simulink model "simulinkm2"  (R2020b)
settings: Solver=VariableStepAuto  StartTime=0.0  StopTime=10.0  RelTol=1e-3
(part 4 of 5)

== matlab function simulinkm2/MATLAB Function3 ==
  data: q input; A_F output; q_dot input; q_double_dot input
  function A_F = forward_acceleration_kinematics(q,q_dot, q_double_dot)
  
     q1 = q(1)
     q2 = q(2)
     q3 = q(3)
     q4 = q(4)
     q5 = q(5)
     q6 = q(6)
     q_double_dot1 = q_double_dot(1) 
     q_double_dot2 = q_double_dot(2) 
     q_double_dot3 = q_double_dot(3) 
     q_double_dot4 = q_double_dot(4) 
     q_double_dot5 = q_double_dot(5) 
     q_double_dot6 = q_double_dot(6)
     q_dot1 = q_dot(1)
     q_dot2 = q_dot(2)
     q_dot3 = q_dot(3)
     q_dot4 = q_dot(4)
     q_dot5 = q_dot(5)
     q_dot6 = q_dot(6)
  
   j_dot = [-q_dot1*((pi*cos((pi*q1)/180))/36 + 10*sin((pi*q5)/180)*((pi*sin((pi*q1)/180)*sin((pi*q4)/180))/180 + (pi*cos((pi*q1)/180)*cos((pi*q2)/180)*cos((pi*q3)/180)*cos((pi*q4)/180))/180 - (pi*cos((pi*q1)/180)*cos((pi*q4)/180)*sin((pi*q2)/180)*sin((pi*q3)/180))/180) + (pi*cos((pi*q1)/180)*cos((pi*q2)/180))/36 + (pi*sin((pi*(q2 + q3))/180)*cos((pi*q1)/180)*cos((pi*q5)/180))/18 + (pi*cos((pi*q1)/180)*cos((pi*q2)/180)*sin((pi*q3)/180))/18 + (pi*cos((pi*q1)/180)*cos((pi*q3)/180)*sin((pi*q2)/180))/18),                                                                                                                                                                                                                                                                                                                                                                                                                                                                                                                                                                                                                                              -q_dot2*cos((pi*q1)/180)*((pi*sin((pi*(q2 + q3))/180))/18 + (pi*cos((pi*q2)/180))/36 + (pi*cos((pi*(q2 + q3))/180)*sin((pi*(q4 + q5))/180))/36 + (pi*sin((pi*(q2 + q3))/180)*cos((pi*q5)/180))/18 - (pi*cos((pi*(q2 + q3))/180)*sin((pi*(q4 - q5))/180))/36),                                                                                                                                                                                                                                                                                                                                                                                                                                                                                                                                                                                 -q_dot3*cos((pi*q1)/180)*((pi*sin((pi*(q2 + q3))/180))/18 + (pi*cos((pi*(q2 + q3))/180)*sin((pi*(q4 + q5))/180))/36 + (pi*sin((pi*(q2 + q3))/180)*cos((pi*q5)/180))/18 - (pi*cos((pi*(q2 + q3))/180)*sin((pi*(q4 - q5))/180))/36),                                                                                                                             -q_dot4*(10*cos((pi*(q2 + q3))/180)*sin((pi*q5)/180)*((pi*cos((pi*q1)/180)*cos((pi*q4)/180))/180 - (pi*sin((pi*q1)/180)*sin((pi*q2)/180)*sin((pi*q3)/180)*sin((pi*q4)/180))/180 + (pi*cos((pi*q2)/180)*cos((pi*q3)/180)*sin((pi*q1)/180)*sin((pi*q4)/180))/180) - sin((pi*(q2 + q3))/180)*sin((pi*q1)/180)*((pi*cos((pi*(q4 + q5))/180)*sin((pi*(q2 + q3))/180))/36 - (pi*sin((pi*(q2 + q3))/180)*cos((pi*(q4 - q5))/180))/36)),                                                                                                                                                                                                                                -q_dot5*((cos((pi*q1)/180)*cos((pi*q4)/180) - sin((pi*q4)/180)*(sin((pi*q1)/180)*sin((pi*q2)/180)*sin((pi*q3)/180) - cos((pi*q2)/180)*cos((pi*q3)/180)*sin((pi*q1)/180)))*((pi*cos((pi*(q4 + q5))/180)*sin((pi*(q2 + q3))/180))/36 + (pi*cos((pi*(q2 + q3))/180)*sin((pi*q5)/180))/18 + (pi*sin((pi*(q2 + q3))/180)*cos((pi*(q4 - q5))/180))/36) + sin((pi*(q2 + q3))/180)*sin((pi*q4)/180)*((pi*cos((pi*q5)/180)*(cos((pi*q1)/180)*sin((pi*q4)/180) - cos((pi*q2)/180)*cos((pi*q3)/180)*cos((pi*q4)/180)*sin((pi*q1)/180) + cos((pi*q4)/180)*sin((pi*q1)/180)*sin((pi*q2)/180)*sin((pi*q3)/180)))/18 + (pi*sin((pi*(q2 + q3))/180)*sin((pi*q1)/180)*sin((pi*q5)/180))/18)), 0;
                   -q_dot1*((pi*sin((pi*q1)/180))/36 - 10*sin((pi*q5)/180)*((pi*cos((pi*q1)/180)*sin((pi*q4)/180))/180 - (pi*cos((pi*q2)/180)*cos((pi*q3)/180)*cos((pi*q4)/180)*sin((pi*q1)/180))/180 + (pi*cos((pi*q4)/180)*sin((pi*q1)/180)*sin((pi*q2)/180)*sin((pi*q3)/180))/180) + (pi*cos((pi*q2)/180)*sin((pi*q1)/180))/36 + (pi*sin((pi*(q2 + q3))/180)*cos((pi*q5)/180)*sin((pi*q1)/180))/18 + (pi*cos((pi*q2)/180)*sin((pi*q1)/180)*sin((pi*q3)/180))/18 + (pi*cos((pi*q3)/180)*sin((pi*q1)/180)*sin((pi*q2)/180))/18),                                                                                                                                                                                                                                                                                                                                                                                                                                                                                                                                                                                                                                              -q_dot2*sin((pi*q1)/180)*((pi*sin((pi*(q2 + q3))/180))/18 + (pi*cos((pi*q2)/180))/36 + (pi*cos((pi*(q2 + q3))/180)*sin((pi*(q4 + q5))/180))/36 + (pi*sin((pi*(q2 + q3))/180)*cos((pi*q5)/180))/18 - (pi*cos((pi*(q2 + q3))/180)*sin((pi*(q4 - q5))/180))/36),                                                                                                                                                                                                                                                                                                                                                                                                                                                                                                                                                                                 -q_dot3*sin((pi*q1)/180)*((pi*sin((pi*(q2 + q3))/180))/18 + (pi*cos((pi*(q2 + q3))/180)*sin((pi*(q4 + q5))/180))/36 + (pi*sin((pi*(q2 + q3))/180)*cos((pi*q5)/180))/18 - (pi*cos((pi*(q2 + q3))/180)*sin((pi*(q4 - q5))/180))/36),                                                                                                                             -q_dot4*(10*cos((pi*(q2 + q3))/180)*sin((pi*q5)/180)*((pi*cos((pi*q4)/180)*sin((pi*q1)/180))/180 - (pi*cos((pi*q1)/180)*cos((pi*q2)/180)*cos((pi*q3)/180)*sin((pi*q4)/180))/180 + (pi*cos((pi*q1)/180)*sin((pi*q2)/180)*sin((pi*q3)/180)*sin((pi*q4)/180))/180) + sin((pi*(q2 + q3))/180)*cos((pi*q1)/180)*((pi*cos((pi*(q4 + q5))/180)*sin((pi*(q2 + q3))/180))/36 - (pi*sin((pi*(q2 + q3))/180)*cos((pi*(q4 - q5))/180))/36)),                                                                                                                                                                                                                                -q_dot5*((sin((pi*q4)/180)*(cos((pi*q1)/180)*sin((pi*q2)/180)*sin((pi*q3)/180) - cos((pi*q1)/180)*cos((pi*q2)/180)*cos((pi*q3)/180)) + cos((pi*q4)/180)*sin((pi*q1)/180))*((pi*cos((pi*(q4 + q5))/180)*sin((pi*(q2 + q3))/180))/36 + (pi*cos((pi*(q2 + q3))/180)*sin((pi*q5)/180))/18 + (pi*sin((pi*(q2 + q3))/180)*cos((pi*(q4 - q5))/180))/36) + sin((pi*(q2 + q3))/180)*sin((pi*q4)/180)*((pi*cos((pi*q5)/180)*(sin((pi*q1)/180)*sin((pi*q4)/180) + cos((pi*q1)/180)*cos((pi*q2)/180)*cos((pi*q3)/180)*cos((pi*q4)/180) - cos((pi*q1)/180)*cos((pi*q4)/180)*sin((pi*q2)/180)*sin((pi*q3)/180)))/18 - (pi*sin((pi*(q2 + q3))/180)*cos((pi*q1)/180)*sin((pi*q5)/180))/18)), 0;
                                                                                                                                                                                                                                                                                                                                                                                                                                                                                                                               0, -q_dot2*(sin((pi*q1)/180)*(10*sin((pi*q5)/180)*((pi*cos((pi*q2)/180)*cos((pi*q4)/180)*sin((pi*q1)/180)*sin((pi*q3)/180))/180 + (pi*cos((pi*q3)/180)*cos((pi*q4)/180)*sin((pi*q1)/180)*sin((pi*q2)/180))/180) + (pi*sin((pi*q1)/180)*sin((pi*q2)/180))/36 - (pi*cos((pi*(q2 + q3))/180)*cos((pi*q5)/180)*sin((pi*q1)/180))/18 - (pi*cos((pi*q2)/180)*cos((pi*q3)/180)*sin((pi*q1)/180))/18 + (pi*sin((pi*q1)/180)*sin((pi*q2)/180)*sin((pi*q3)/180))/18) + cos((pi*q1)/180)*(10*sin((pi*q5)/180)*((pi*cos((pi*q1)/180)*cos((pi*q2)/180)*cos((pi*q4)/180)*sin((pi*q3)/180))/180 + (pi*cos((pi*q1)/180)*cos((pi*q3)/180)*cos((pi*q4)/180)*sin((pi*q2)/180))/180) + (pi*cos((pi*q1)/180)*sin((pi*q2)/180))/36 - (pi*cos((pi*(q2 + q3))/180)*cos((pi*q1)/180)*cos((pi*q5)/180))/18 - (pi*cos((pi*q1)/180)*cos((pi*q2)/180)*cos((pi*q3)/180))/18 + (pi*cos((pi*q1)/180)*sin((pi*q2)/180)*sin((pi*q3)/180))/18)), -q_dot3*(sin((pi*q1)/180)*(10*sin((pi*q5)/180)*((pi*cos((pi*q2)/180)*cos((pi*q4)/180)*sin((pi*q1)/180)*sin((pi*q3)/180))/180 + (pi*cos((pi*q3)/180)*cos((pi*q4)/180)*sin((pi*q1)/180)*sin((pi*q2)/180))/180) - (pi*cos((pi*(q2 + q3))/180)*cos((pi*q5)/180)*sin((pi*q1)/180))/18 - (pi*cos((pi*q2)/180)*cos((pi*q3)/180)*sin((pi*q1)/180))/18 + (pi*sin((pi*q1)/180)*sin((pi*q2)/180)*sin((pi*q3)/180))/18) + cos((pi*q1)/180)*(10*sin((pi*q5)/180)*((pi*cos((pi*q1)/180)*cos((pi*q2)/180)*cos((pi*q4)/180)*sin((pi*q3)/180))/180 + (pi*cos((pi*q1)/180)*cos((pi*q3)/180)*cos((pi*q4)/180)*sin((pi*q2)/180))/180) - (pi*cos((pi*(q2 + q3))/180)*cos((pi*q1)/180)*cos((pi*q5)/180))/18 - (pi*cos((pi*q1)/180)*cos((pi*q2)/180)*cos((pi*q3)/180))/18 + (pi*cos((pi*q1)/180)*sin((pi*q2)/180)*sin((pi*q3)/180))/18)), -q_dot4*(10*sin((pi*(q2 + q3))/180)*cos((pi*q1)/180)*sin((pi*q5)/180)*((pi*cos((pi*q1)/180)*cos((pi*q4)/180))/180 - (pi*sin((pi*q1)/180)*sin((pi*q2)/180)*sin((pi*q3)/180)*sin((pi*q4)/180))/180 + (pi*cos((pi*q2)/180)*cos((pi*q3)/180)*sin((pi*q1)/180)*sin((pi*q4)/180))/180) + 10*sin((pi*(q2 + q3))/180)*sin((pi*q1)/180)*sin((pi*q5)/180)*((pi*cos((pi*q4)/180)*sin((pi*q1)/180))/180 - (pi*cos((pi*q1)/180)*cos((pi*q2)/180)*cos((pi*q3)/180)*sin((pi*q4)/180))/180 + (pi*cos((pi*q1)/180)*sin((pi*q2)/180)*sin((pi*q3)/180)*sin((pi*q4)/180))/180)), q_dot5*((cos((pi*q1)/180)*cos((pi*q4)/180) - sin((pi*q4)/180)*(sin((pi*q1)/180)*sin((pi*q2)/180)*sin((pi*q3)/180) - cos((pi*q2)/180)*cos((pi*q3)/180)*sin((pi*q1)/180)))*((pi*cos((pi*q5)/180)*(sin((pi*q1)/180)*sin((pi*q4)/180) + cos((pi*q1)/180)*cos((pi*q2)/180)*cos((pi*q3)/180)*cos((pi*q4)/180) - cos((pi*q1)/180)*cos((pi*q4)/180)*sin((pi*q2)/180)*sin((pi*q3)/180)))/18 - (pi*sin((pi*(q2 + q3))/180)*cos((pi*q1)/180)*sin((pi*q5)/180))/18) - (sin((pi*q4)/180)*(cos((pi*q1)/180)*sin((pi*q2)/180)*sin((pi*q3)/180) - cos((pi*q1)/180)*cos((pi*q2)/180)*cos((pi*q3)/180)) + cos((pi*q4)/180)*sin((pi*q1)/180))*((pi*cos((pi*q5)/180)*(cos((pi*q1)/180)*sin((pi*q4)/180) - cos((pi*q2)/180)*cos((pi*q3)/180)*cos((pi*q4)/180)*sin((pi*q1)/180) + cos((pi*q4)/180)*sin((pi*q1)/180)*sin((pi*q2)/180)*sin((pi*q3)/180)))/18 + (pi*sin((pi*(q2 + q3))/180)*sin((pi*q1)/180)*sin((pi*q5)/180))/18)), 0;
                                                                                                                                                                                                                                                                                                                                                                                                                                                                                                                               0,                                                                                                                                                                                                                                                                                                                                                                                                                                                                                                                                                                                                                                                                                                                                                                                                                                                                                                         0,                                                                                                                                                                                                                                                                                                                                                                                                                                                                                                                                                                                                                                                                                                                                                                                                                 0,                                                                                                                                                                                                                                                                                                                                                                                                                                                                                                                                                           0,                                                                                                                                                                                                                                                                                                                                                                                                                                                                                                                                                                                                                                                                                                                                                                                                                                                                                                          0, 0;
                                                                                                                                                                                                                                                                                                                                                                                                                                                                                                                               0,                                                                                                                                                                                                                                                                                                                                                                                                                                                                                                                                                                                                                                                                                                                                                                                                                                                                                                         0,                                                                                                                                                                                                                                                                                                                                                                                                                                                                                                                                                                                                                                                                                                                                                                                                                 0,                                                                                                                                                                                                                                                                                                                                                                                                                                                                                                                                                           0,                                                                                                                                                                                                                                                                                                                                                                                                                                                                                                                                                                                                                                                                                                                                                                                                                                                                                                          0, 0;
                                                                                                                                                                                                                                                                                                                                                                                                                                                                                                                               0,                                                                                                                                                                                                                                                                                                                                                                                                                                                                                                                                                                                                                                                                                                                                                                                                                                                                                                         0,                                                                                                                                                                                                                                                                                                                                                                                                                                                                                                                                                                                                                                                                                                                                                                                                                 0,                                                                                                                                                                                                                                                                                                                                                                                                                                                                                                                                                           0,                                                                                                                                                                                                                                                                                                                                                                                                                                                                                                                                                                                                                                                                                                                                                                                                                                                                                                          0, 0]
                                      
   J =[10*sin((pi*q5)/180)*(cos((pi*q1)/180)*sin((pi*q4)/180) - cos((pi*q2)/180)*cos((pi*q3)/180)*cos((pi*q4)/180)*sin((pi*q1)/180) + cos((pi*q4)/180)*sin((pi*q1)/180)*sin((pi*q2)/180)*sin((pi*q3)/180)) - 5*cos((pi*q2)/180)*sin((pi*q1)/180) - 5*sin((pi*q1)/180) - 10*cos((pi*q2)/180)*sin((pi*q1)/180)*sin((pi*q3)/180) - 10*cos((pi*q3)/180)*sin((pi*q1)/180)*sin((pi*q2)/180) - 10*sin((pi*(q2 + q3))/180)*cos((pi*q5)/180)*sin((pi*q1)/180),                                                                                                                                                                                                                                                                                                                                                                                                                                                                                                                                                                                                                                                                  cos((pi*q1)/180)*(10*cos((pi*(q2 + q3))/180) - 5*sin((pi*q2)/180) - 5*sin((pi*(q2 + q3))/180)*sin((pi*(q4 + q5))/180) + 10*cos((pi*(q2 + q3))/180)*cos((pi*q5)/180) + 5*sin((pi*(q2 + q3))/180)*sin((pi*(q4 - q5))/180)),                                                                                                                                                                                                                                                                                                                                                                                                                                                                                                                                                                                                                                                                                                                                                                                                                         cos((pi*q1)/180)*(10*cos((pi*(q2 + q3))/180) - 5*sin((pi*(q2 + q3))/180)*sin((pi*(q4 + q5))/180) + 10*cos((pi*(q2 + q3))/180)*cos((pi*q5)/180) + 5*sin((pi*(q2 + q3))/180)*sin((pi*(q4 - q5))/180)),                                                                                                                                                                                                                                                                                                                           cos((pi*(q2 + q3))/180)*(5*sin((pi*q1)/180) + 5*cos((pi*q2)/180)*sin((pi*q1)/180) - 5*sin((pi*q1)/180)*(cos((pi*q2)/180) + 1) - 10*sin((pi*q5)/180)*(cos((pi*q1)/180)*sin((pi*q4)/180) - cos((pi*q2)/180)*cos((pi*q3)/180)*cos((pi*q4)/180)*sin((pi*q1)/180) + cos((pi*q4)/180)*sin((pi*q1)/180)*sin((pi*q2)/180)*sin((pi*q3)/180)) + 10*cos((pi*q2)/180)*sin((pi*q1)/180)*sin((pi*q3)/180) + 10*cos((pi*q3)/180)*sin((pi*q1)/180)*sin((pi*q2)/180) + 10*sin((pi*(q2 + q3))/180)*cos((pi*q5)/180)*sin((pi*q1)/180)) - sin((pi*(q2 + q3))/180)*sin((pi*q1)/180)*(10*cos((pi*(q2 + q3))/180) - 5*sin((pi*(q2 + q3))/180)*sin((pi*(q4 + q5))/180) + 10*cos((pi*(q2 + q3))/180)*cos((pi*q5)/180) + 5*sin((pi*(q2 + q3))/180)*sin((pi*(q4 - q5))/180)),                                                                                                                                                                                                                                                                                                                                                                                                                                                                                           (cos((pi*q1)/180)*cos((pi*q4)/180) - sin((pi*q4)/180)*(sin((pi*q1)/180)*sin((pi*q2)/180)*sin((pi*q3)/180) - cos((pi*q2)/180)*cos((pi*q3)/180)*sin((pi*q1)/180)))*(10*cos((pi*(q2 + q3))/180)*cos((pi*q5)/180) - 5*sin((pi*(q2 + q3))/180)*sin((pi*(q4 + q5))/180) + 5*sin((pi*(q2 + q3))/180)*sin((pi*(q4 - q5))/180)) + sin((pi*(q2 + q3))/180)*sin((pi*q4)/180)*(5*sin((pi*q1)/180) + 5*cos((pi*q2)/180)*sin((pi*q1)/180) - 5*sin((pi*q1)/180)*(2*sin((pi*(q2 + q3))/180) + cos((pi*q2)/180) + 1) - 10*sin((pi*q5)/180)*(cos((pi*q1)/180)*sin((pi*q4)/180) - cos((pi*q2)/180)*cos((pi*q3)/180)*cos((pi*q4)/180)*sin((pi*q1)/180) + cos((pi*q4)/180)*sin((pi*q1)/180)*sin((pi*q2)/180)*sin((pi*q3)/180)) + 10*cos((pi*q2)/180)*sin((pi*q1)/180)*sin((pi*q3)/180) + 10*cos((pi*q3)/180)*sin((pi*q1)/180)*sin((pi*q2)/180) + 10*sin((pi*(q2 + q3))/180)*cos((pi*q5)/180)*sin((pi*q1)/180)),                                                                                                                                                                                                                                                                                                                                                                                                                                                                                                                                                                             (cos((pi*(q2 + q3))/180)*cos((pi*q5)/180) - sin((pi*(q2 + q3))/180)*cos((pi*q4)/180)*sin((pi*q5)/180))*(5*sin((pi*q1)/180) + 5*cos((pi*q2)/180)*sin((pi*q1)/180) - 5*sin((pi*q1)/180)*(2*sin((pi*(q2 + q3))/180) + cos((pi*q2)/180) + 1) - 10*sin((pi*q5)/180)*(cos((pi*q1)/180)*sin((pi*q4)/180) - cos((pi*q2)/180)*cos((pi*q3)/180)*cos((pi*q4)/180)*sin((pi*q1)/180) + cos((pi*q4)/180)*sin((pi*q1)/180)*sin((pi*q2)/180)*sin((pi*q3)/180)) + 10*cos((pi*q2)/180)*sin((pi*q1)/180)*sin((pi*q3)/180) + 10*cos((pi*q3)/180)*sin((pi*q1)/180)*sin((pi*q2)/180) + 10*sin((pi*(q2 + q3))/180)*cos((pi*q5)/180)*sin((pi*q1)/180)) + (sin((pi*q5)/180)*(cos((pi*q4)/180)*(sin((pi*q1)/180)*sin((pi*q2)/180)*sin((pi*q3)/180) - cos((pi*q2)/180)*cos((pi*q3)/180)*sin((pi*q1)/180)) + cos((pi*q1)/180)*sin((pi*q4)/180)) - cos((pi*q5)/180)*(cos((pi*q2)/180)*sin((pi*q1)/180)*sin((pi*q3)/180) + cos((pi*q3)/180)*sin((pi*q1)/180)*sin((pi*q2)/180)))*(10*cos((pi*(q2 + q3))/180)*cos((pi*q5)/180) - 5*sin((pi*(q2 + q3))/180)*sin((pi*(q4 + q5))/180) + 5*sin((pi*(q2 + q3))/180)*sin((pi*(q4 - q5))/180));
5*cos((pi*q1)/180) + 5*cos((pi*q1)/180)*cos((pi*q2)/180) + 10*sin((pi*q5)/180)*(sin((pi*q1)/180)*sin((pi*q4)/180) + cos((pi*q1)/180)*cos((pi*q2)/180)*cos((pi*q3)/180)*cos((pi*q4)/180) - cos((pi*q1)/180)*cos((pi*q4)/180)*sin((pi*q2)/180)*sin((pi*q3)/180)) + 10*sin((pi*(q2 + q3))/180)*cos((pi*q1)/180)*cos((pi*q5)/180) + 10*cos((pi*q1)/180)*cos((pi*q2)/180)*sin((pi*q3)/180) + 10*cos((pi*q1)/180)*cos((pi*q3)/180)*sin((pi*q2)/180),                                                                                                                                                                                                                                                                                                                                                                                                                                                                                                                                                                                                                                                                  sin((pi*q1)/180)*(10*cos((pi*(q2 + q3))/180) - 5*sin((pi*q2)/180) - 5*sin((pi*(q2 + q3))/180)*sin((pi*(q4 + q5))/180) + 10*cos((pi*(q2 + q3))/180)*cos((pi*q5)/180) + 5*sin((pi*(q2 + q3))/180)*sin((pi*(q4 - q5))/180)),                                                                                                                                                                                                                                                                                                                                                                                                                                                                                                                                                                                                                                                                                                                                                                                                                         sin((pi*q1)/180)*(10*cos((pi*(q2 + q3))/180) - 5*sin((pi*(q2 + q3))/180)*sin((pi*(q4 + q5))/180) + 10*cos((pi*(q2 + q3))/180)*cos((pi*q5)/180) + 5*sin((pi*(q2 + q3))/180)*sin((pi*(q4 - q5))/180)),                                                                                                                                                                                                                                                                                                                           sin((pi*(q2 + q3))/180)*cos((pi*q1)/180)*(10*cos((pi*(q2 + q3))/180) - 5*sin((pi*(q2 + q3))/180)*sin((pi*(q4 + q5))/180) + 10*cos((pi*(q2 + q3))/180)*cos((pi*q5)/180) + 5*sin((pi*(q2 + q3))/180)*sin((pi*(q4 - q5))/180)) - cos((pi*(q2 + q3))/180)*(5*cos((pi*q1)/180) + 5*cos((pi*q1)/180)*cos((pi*q2)/180) - 5*cos((pi*q1)/180)*(cos((pi*q2)/180) + 1) + 10*sin((pi*q5)/180)*(sin((pi*q1)/180)*sin((pi*q4)/180) + cos((pi*q1)/180)*cos((pi*q2)/180)*cos((pi*q3)/180)*cos((pi*q4)/180) - cos((pi*q1)/180)*cos((pi*q4)/180)*sin((pi*q2)/180)*sin((pi*q3)/180)) + 10*sin((pi*(q2 + q3))/180)*cos((pi*q1)/180)*cos((pi*q5)/180) + 10*cos((pi*q1)/180)*cos((pi*q2)/180)*sin((pi*q3)/180) + 10*cos((pi*q1)/180)*cos((pi*q3)/180)*sin((pi*q2)/180)),                                                                                                                                                                                                                                                                                                                                                                                                                                                                                           (sin((pi*q4)/180)*(cos((pi*q1)/180)*sin((pi*q2)/180)*sin((pi*q3)/180) - cos((pi*q1)/180)*cos((pi*q2)/180)*cos((pi*q3)/180)) + cos((pi*q4)/180)*sin((pi*q1)/180))*(10*cos((pi*(q2 + q3))/180)*cos((pi*q5)/180) - 5*sin((pi*(q2 + q3))/180)*sin((pi*(q4 + q5))/180) + 5*sin((pi*(q2 + q3))/180)*sin((pi*(q4 - q5))/180)) - sin((pi*(q2 + q3))/180)*sin((pi*q4)/180)*(5*cos((pi*q1)/180) + 5*cos((pi*q1)/180)*cos((pi*q2)/180) - 5*cos((pi*q1)/180)*(2*sin((pi*(q2 + q3))/180) + cos((pi*q2)/180) + 1) + 10*sin((pi*q5)/180)*(sin((pi*q1)/180)*sin((pi*q4)/180) + cos((pi*q1)/180)*cos((pi*q2)/180)*cos((pi*q3)/180)*cos((pi*q4)/180) - cos((pi*q1)/180)*cos((pi*q4)/180)*sin((pi*q2)/180)*sin((pi*q3)/180)) + 10*sin((pi*(q2 + q3))/180)*cos((pi*q1)/180)*cos((pi*q5)/180) + 10*cos((pi*q1)/180)*cos((pi*q2)/180)*sin((pi*q3)/180) + 10*cos((pi*q1)/180)*cos((pi*q3)/180)*sin((pi*q2)/180)),                                                                                                                                                                                                                                                                                                                                                                                                                                                                                                                                                                           - (sin((pi*q5)/180)*(cos((pi*q4)/180)*(cos((pi*q1)/180)*sin((pi*q2)/180)*sin((pi*q3)/180) - cos((pi*q1)/180)*cos((pi*q2)/180)*cos((pi*q3)/180)) - sin((pi*q1)/180)*sin((pi*q4)/180)) - cos((pi*q5)/180)*(cos((pi*q1)/180)*cos((pi*q2)/180)*sin((pi*q3)/180) + cos((pi*q1)/180)*cos((pi*q3)/180)*sin((pi*q2)/180)))*(10*cos((pi*(q2 + q3))/180)*cos((pi*q5)/180) - 5*sin((pi*(q2 + q3))/180)*sin((pi*(q4 + q5))/180) + 5*sin((pi*(q2 + q3))/180)*sin((pi*(q4 - q5))/180)) - (cos((pi*(q2 + q3))/180)*cos((pi*q5)/180) - sin((pi*(q2 + q3))/180)*cos((pi*q4)/180)*sin((pi*q5)/180))*(5*cos((pi*q1)/180) + 5*cos((pi*q1)/180)*cos((pi*q2)/180) - 5*cos((pi*q1)/180)*(2*sin((pi*(q2 + q3))/180) + cos((pi*q2)/180) + 1) + 10*sin((pi*q5)/180)*(sin((pi*q1)/180)*sin((pi*q4)/180) + cos((pi*q1)/180)*cos((pi*q2)/180)*cos((pi*q3)/180)*cos((pi*q4)/180) - cos((pi*q1)/180)*cos((pi*q4)/180)*sin((pi*q2)/180)*sin((pi*q3)/180)) + 10*sin((pi*(q2 + q3))/180)*cos((pi*q1)/180)*cos((pi*q5)/180) + 10*cos((pi*q1)/180)*cos((pi*q2)/180)*sin((pi*q3)/180) + 10*cos((pi*q1)/180)*cos((pi*q3)/180)*sin((pi*q2)/180));
                                                                                                                                                                                                                                                                                                                                                                                                                                            0, cos((pi*q1)/180)*(5*cos((pi*q1)/180)*cos((pi*q2)/180) + 10*sin((pi*q5)/180)*(sin((pi*q1)/180)*sin((pi*q4)/180) + cos((pi*q1)/180)*cos((pi*q2)/180)*cos((pi*q3)/180)*cos((pi*q4)/180) - cos((pi*q1)/180)*cos((pi*q4)/180)*sin((pi*q2)/180)*sin((pi*q3)/180)) + 10*sin((pi*(q2 + q3))/180)*cos((pi*q1)/180)*cos((pi*q5)/180) + 10*cos((pi*q1)/180)*cos((pi*q2)/180)*sin((pi*q3)/180) + 10*cos((pi*q1)/180)*cos((pi*q3)/180)*sin((pi*q2)/180)) + sin((pi*q1)/180)*(5*cos((pi*q2)/180)*sin((pi*q1)/180) - 10*sin((pi*q5)/180)*(cos((pi*q1)/180)*sin((pi*q4)/180) - cos((pi*q2)/180)*cos((pi*q3)/180)*cos((pi*q4)/180)*sin((pi*q1)/180) + cos((pi*q4)/180)*sin((pi*q1)/180)*sin((pi*q2)/180)*sin((pi*q3)/180)) + 10*cos((pi*q2)/180)*sin((pi*q1)/180)*sin((pi*q3)/180) + 10*cos((pi*q3)/180)*sin((pi*q1)/180)*sin((pi*q2)/180) + 10*sin((pi*(q2 + q3))/180)*cos((pi*q5)/180)*sin((pi*q1)/180)), sin((pi*q1)/180)*(5*sin((pi*q1)/180) + 5*cos((pi*q2)/180)*sin((pi*q1)/180) - 5*sin((pi*q1)/180)*(cos((pi*q2)/180) + 1) - 10*sin((pi*q5)/180)*(cos((pi*q1)/180)*sin((pi*q4)/180) - cos((pi*q2)/180)*cos((pi*q3)/180)*cos((pi*q4)/180)*sin((pi*q1)/180) + cos((pi*q4)/180)*sin((pi*q1)/180)*sin((pi*q2)/180)*sin((pi*q3)/180)) + 10*cos((pi*q2)/180)*sin((pi*q1)/180)*sin((pi*q3)/180) + 10*cos((pi*q3)/180)*sin((pi*q1)/180)*sin((pi*q2)/180) + 10*sin((pi*(q2 + q3))/180)*cos((pi*q5)/180)*sin((pi*q1)/180)) + cos((pi*q1)/180)*(5*cos((pi*q1)/180) + 5*cos((pi*q1)/180)*cos((pi*q2)/180) - 5*cos((pi*q1)/180)*(cos((pi*q2)/180) + 1) + 10*sin((pi*q5)/180)*(sin((pi*q1)/180)*sin((pi*q4)/180) + cos((pi*q1)/180)*cos((pi*q2)/180)*cos((pi*q3)/180)*cos((pi*q4)/180) - cos((pi*q1)/180)*cos((pi*q4)/180)*sin((pi*q2)/180)*sin((pi*q3)/180)) + 10*sin((pi*(q2 + q3))/180)*cos((pi*q1)/180)*cos((pi*q5)/180) + 10*cos((pi*q1)/180)*cos((pi*q2)/180)*sin((pi*q3)/180) + 10*cos((pi*q1)/180)*cos((pi*q3)/180)*sin((pi*q2)/180)), sin((pi*(q2 + q3))/180)*cos((pi*q1)/180)*(5*sin((pi*q1)/180) + 5*cos((pi*q2)/180)*sin((pi*q1)/180) - 5*sin((pi*q1)/180)*(cos((pi*q2)/180) + 1) - 10*sin((pi*q5)/180)*(cos((pi*q1)/180)*sin((pi*q4)/180) - cos((pi*q2)/180)*cos((pi*q3)/180)*cos((pi*q4)/180)*sin((pi*q1)/180) + cos((pi*q4)/180)*sin((pi*q1)/180)*sin((pi*q2)/180)*sin((pi*q3)/180)) + 10*cos((pi*q2)/180)*sin((pi*q1)/180)*sin((pi*q3)/180) + 10*cos((pi*q3)/180)*sin((pi*q1)/180)*sin((pi*q2)/180) + 10*sin((pi*(q2 + q3))/180)*cos((pi*q5)/180)*sin((pi*q1)/180)) - sin((pi*(q2 + q3))/180)*sin((pi*q1)/180)*(5*cos((pi*q1)/180) + 5*cos((pi*q1)/180)*cos((pi*q2)/180) - 5*cos((pi*q1)/180)*(cos((pi*q2)/180) + 1) + 10*sin((pi*q5)/180)*(sin((pi*q1)/180)*sin((pi*q4)/180) + cos((pi*q1)/180)*cos((pi*q2)/180)*cos((pi*q3)/180)*cos((pi*q4)/180) - cos((pi*q1)/180)*cos((pi*q4)/180)*sin((pi*q2)/180)*sin((pi*q3)/180)) + 10*sin((pi*(q2 + q3))/180)*cos((pi*q1)/180)*cos((pi*q5)/180) + 10*cos((pi*q1)/180)*cos((pi*q2)/180)*sin((pi*q3)/180) + 10*cos((pi*q1)/180)*cos((pi*q3)/180)*sin((pi*q2)/180)), (cos((pi*q1)/180)*cos((pi*q4)/180) - sin((pi*q4)/180)*(sin((pi*q1)/180)*sin((pi*q2)/180)*sin((pi*q3)/180) - cos((pi*q2)/180)*cos((pi*q3)/180)*sin((pi*q1)/180)))*(5*cos((pi*q1)/180) + 5*cos((pi*q1)/180)*cos((pi*q2)/180) - 5*cos((pi*q1)/180)*(2*sin((pi*(q2 + q3))/180) + cos((pi*q2)/180) + 1) + 10*sin((pi*q5)/180)*(sin((pi*q1)/180)*sin((pi*q4)/180) + cos((pi*q1)/180)*cos((pi*q2)/180)*cos((pi*q3)/180)*cos((pi*q4)/180) - cos((pi*q1)/180)*cos((pi*q4)/180)*sin((pi*q2)/180)*sin((pi*q3)/180)) + 10*sin((pi*(q2 + q3))/180)*cos((pi*q1)/180)*cos((pi*q5)/180) + 10*cos((pi*q1)/180)*cos((pi*q2)/180)*sin((pi*q3)/180) + 10*cos((pi*q1)/180)*cos((pi*q3)/180)*sin((pi*q2)/180)) + (sin((pi*q4)/180)*(cos((pi*q1)/180)*sin((pi*q2)/180)*sin((pi*q3)/180) - cos((pi*q1)/180)*cos((pi*q2)/180)*cos((pi*q3)/180)) + cos((pi*q4)/180)*sin((pi*q1)/180))*(5*sin((pi*q1)/180) + 5*cos((pi*q2)/180)*sin((pi*q1)/180) - 5*sin((pi*q1)/180)*(2*sin((pi*(q2 + q3))/180) + cos((pi*q2)/180) + 1) - 10*sin((pi*q5)/180)*(cos((pi*q1)/180)*sin((pi*q4)/180) - cos((pi*q2)/180)*cos((pi*q3)/180)*cos((pi*q4)/180)*sin((pi*q1)/180) + cos((pi*q4)/180)*sin((pi*q1)/180)*sin((pi*q2)/180)*sin((pi*q3)/180)) + 10*cos((pi*q2)/180)*sin((pi*q1)/180)*sin((pi*q3)/180) + 10*cos((pi*q3)/180)*sin((pi*q1)/180)*sin((pi*q2)/180) + 10*sin((pi*(q2 + q3))/180)*cos((pi*q5)/180)*sin((pi*q1)/180)), (sin((pi*q5)/180)*(cos((pi*q4)/180)*(sin((pi*q1)/180)*sin((pi*q2)/180)*sin((pi*q3)/180) - cos((pi*q2)/180)*cos((pi*q3)/180)*sin((pi*q1)/180)) + cos((pi*q1)/180)*sin((pi*q4)/180)) - cos((pi*q5)/180)*(cos((pi*q2)/180)*sin((pi*q1)/180)*sin((pi*q3)/180) + cos((pi*q3)/180)*sin((pi*q1)/180)*sin((pi*q2)/180)))*(5*cos((pi*q1)/180) + 5*cos((pi*q1)/180)*cos((pi*q2)/180) - 5*cos((pi*q1)/180)*(2*sin((pi*(q2 + q3))/180) + cos((pi*q2)/180) + 1) + 10*sin((pi*q5)/180)*(sin((pi*q1)/180)*sin((pi*q4)/180) + cos((pi*q1)/180)*cos((pi*q2)/180)*cos((pi*q3)/180)*cos((pi*q4)/180) - cos((pi*q1)/180)*cos((pi*q4)/180)*sin((pi*q2)/180)*sin((pi*q3)/180)) + 10*sin((pi*(q2 + q3))/180)*cos((pi*q1)/180)*cos((pi*q5)/180) + 10*cos((pi*q1)/180)*cos((pi*q2)/180)*sin((pi*q3)/180) + 10*cos((pi*q1)/180)*cos((pi*q3)/180)*sin((pi*q2)/180)) - (sin((pi*q5)/180)*(cos((pi*q4)/180)*(cos((pi*q1)/180)*sin((pi*q2)/180)*sin((pi*q3)/180) - cos((pi*q1)/180)*cos((pi*q2)/180)*cos((pi*q3)/180)) - sin((pi*q1)/180)*sin((pi*q4)/180)) - cos((pi*q5)/180)*(cos((pi*q1)/180)*cos((pi*q2)/180)*sin((pi*q3)/180) + cos((pi*q1)/180)*cos((pi*q3)/180)*sin((pi*q2)/180)))*(5*sin((pi*q1)/180) + 5*cos((pi*q2)/180)*sin((pi*q1)/180) - 5*sin((pi*q1)/180)*(2*sin((pi*(q2 + q3))/180) + cos((pi*q2)/180) + 1) - 10*sin((pi*q5)/180)*(cos((pi*q1)/180)*sin((pi*q4)/180) - cos((pi*q2)/180)*cos((pi*q3)/180)*cos((pi*q4)/180)*sin((pi*q1)/180) + cos((pi*q4)/180)*sin((pi*q1)/180)*sin((pi*q2)/180)*sin((pi*q3)/180)) + 10*cos((pi*q2)/180)*sin((pi*q1)/180)*sin((pi*q3)/180) + 10*cos((pi*q3)/180)*sin((pi*q1)/180)*sin((pi*q2)/180) + 10*sin((pi*(q2 + q3))/180)*cos((pi*q5)/180)*sin((pi*q1)/180));
                                                                                                                                                                                                                                                                                                                                                                                                                                            0,                                                                                                                                                                                                                                                                                                                                                                                                                                                                                                                                                                                                                                                                                                                                                                                                                                                                          sin((pi*q1)/180),                                                                                                                                                                                                                                                                                                                                                                                                                                                                                                                                                                                                                                                                                                                                                                                                                                                                                                                                                                                                            sin((pi*q1)/180),                                                                                                                                                                                                                                                                                                                                                                                                                                                                                                                                                                                                                                                                                                                                                                                                                                                                                                                                                                                                                                    sin((pi*(q2 + q3))/180)*cos((pi*q1)/180),                                                                                                                                                                                                                                                                                                                                                                                                                                                                                                                                                                                                                                                                                                                                                                                                                                                                                                                                                                                                                                                                                                                                                                                                                      sin((pi*q4)/180)*(cos((pi*q1)/180)*sin((pi*q2)/180)*sin((pi*q3)/180) - cos((pi*q1)/180)*cos((pi*q2)/180)*cos((pi*q3)/180)) + cos((pi*q4)/180)*sin((pi*q1)/180),                                                                                                                                                                                                                                                                                                                                                                                                                                                                                                                                                                                                                                                                                                                                                                                                                                                                                                                                                                                                                                                                                                                                                                                                                                                                                                                                                                      cos((pi*q5)/180)*(cos((pi*q1)/180)*cos((pi*q2)/180)*sin((pi*q3)/180) + cos((pi*q1)/180)*cos((pi*q3)/180)*sin((pi*q2)/180)) - sin((pi*q5)/180)*(cos((pi*q4)/180)*(cos((pi*q1)/180)*sin((pi*q2)/180)*sin((pi*q3)/180) - cos((pi*q1)/180)*cos((pi*q2)/180)*cos((pi*q3)/180)) - sin((pi*q1)/180)*sin((pi*q4)/180));
                                                                                                                                                                                                                                                                                                                                                                                                                                            0,                                                                                                                                                                                                                                                                                                                                                                                                                                                                                                                                                                                                                                                                                                                                                                                                                                                                         -cos((pi*q1)/180),                                                                                                                                                                                                                                                                                                                                                                                                                                                                                                                                                                                                                                                                                                                                                                                                                                                                                                                                                                                                           -cos((pi*q1)/180),                                                                                                                                                                                                                                                                                                                                                                                                                                                                                                                                                                                                                                                                                                                                                                                                                                                                                                                                                                                                                                    sin((pi*(q2 + q3))/180)*sin((pi*q1)/180),                                                                                                                                                                                                                                                                                                                                                                                                                                                                                                                                                                                                                                                                                                                                                                                                                                                                                                                                                                                                                                                                                                                                                                                                                      sin((pi*q4)/180)*(sin((pi*q1)/180)*sin((pi*q2)/180)*sin((pi*q3)/180) - cos((pi*q2)/180)*cos((pi*q3)/180)*sin((pi*q1)/180)) - cos((pi*q1)/180)*cos((pi*q4)/180),                                                                                                                                                                                                                                                                                                                                                                                                                                                                                                                                                                                                                                                                                                                                                                                                                                                                                                                                                                                                                                                                                                                                                                                                                                                                                                                                                                      cos((pi*q5)/180)*(cos((pi*q2)/180)*sin((pi*q1)/180)*sin((pi*q3)/180) + cos((pi*q3)/180)*sin((pi*q1)/180)*sin((pi*q2)/180)) - sin((pi*q5)/180)*(cos((pi*q4)/180)*(sin((pi*q1)/180)*sin((pi*q2)/180)*sin((pi*q3)/180) - cos((pi*q2)/180)*cos((pi*q3)/180)*sin((pi*q1)/180)) + cos((pi*q1)/180)*sin((pi*q4)/180));
                                                                                                                                                                                                                                                                                                                                                                                                                                            1,                                                                                                                                                                                                                                                                                                                                                                                                                                                                                                                                                                                                                                                                                                                                                                                                                                                                                         0,                                                                                                                                                                                                                                                                                                                                                                                                                                                                                                                                                                                                                                                                                                                                                                                                                                                                                                                                                                                                                           0,                                                                                                                                                                                                                                                                                                                                                                                                                                                                                                                                                                                                                                                                                                                                                                                                                                                                                                                                                                                                                                                    -cos((pi*(q2 + q3))/180),                                                                                                                                                                                                                                                                                                                                                                                                                                                                                                                                                                                                                                                                                                                                                                                                                                                                                                                                                                                                                                                                                                                                                                                                                                                                                                                                           -sin((pi*(q2 + q3))/180)*sin((pi*q4)/180),                                                                                                                                                                                                                                                                                                                                                                                                                                                                                                                                                                                                                                                                                                                                                                                                                                                                                                                                                                                                                                                                                                                                                                                                                                                                                                                                                                                                                                                                                                                                                                                sin((pi*(q2 + q3))/180)*cos((pi*q4)/180)*sin((pi*q5)/180) - cos((pi*(q2 + q3))/180)*cos((pi*q5)/180)]
 
    
  
   
    A = j_dot * q_dot 
    B = J * q_double_dot 
    A_F = A + B
  end
